simulink model "cmld_1m_vt"  (R2025b)
settings: Solver=ode23tb  StartTime=0.0  StopTime=12  MaxStep=5e-4  RelTol=1e-3
PreLoadFcn:
  | % --- generated CMLD self-contained defaults (cmld_params_for recipe, P=2405 MW baseline) ---
  | MotorA_Nom=[487413333.333333 11000 50]; MotorA_Stator=[0.02 0.072]; MotorA_Rotor=[0.05955 0.04937]; MotorA_Lm=1.728; MotorA_Mech=[0.1 0 2]; MotorA_Pmec=365560000; MotorA_Tm=0.786871368; MotorA_IC=[0.046858189966907 0 0 0 0 0 -120 120];
  | MotorB_Nom=[532306666.666667 11000 50]; MotorB_Stator=[0.03 0.114]; MotorB_Rotor=[0.0281 0.07959]; MotorB_Lm=1.686; MotorB_Mech=[0.5 0 2]; MotorB_Pmec=399230000; MotorB_Tm=0.7665097973; MotorB_IC=[0.0215389253032176 0 0 0 0 0 -120 120];
  | MotorC_Nom=[413660000 11000 50]; MotorC_Stator=[0.03 0.114]; MotorC_Rotor=[0.0281 0.07959]; MotorC_Lm=1.686; MotorC_Mech=[0.1 0 2]; MotorC_Pmec=310245000; MotorC_Tm=0.7665097973; MotorC_IC=[0.0215389253032176 0 0 0 0 0 -120 120];
  | CMLD_ElecP=810485000; P0=409480000; Q0=103896000; Pfrq=1.0;
  | CapC=0.037092; Fb_head=0.5;
undefined symbols (not defined in the file): dist_dP, dist_time, k_droop_f_g1, kt_hp, kt_lp, Lg_n1, M_g1, Motor_Tm, P_ref_g1, Rg_n1, Scc1, t_rh, theta_g0, Un1, Vpeak_g1, w_g1
libraries: spsControlledVoltageSourceLib x3, spsGroundLib x3, spsSeriesRLCBranchLib x3, spsThreePhaseParallelRLCBranchLib x2, spsThreePhaseParallelRLCLoadLib x1, spsThreePhaseSeriesRLCBranchLib x1, spsAsynchronousMachinepuUnitsLib x1, spsThreePhaseDynamicLoadLib x1, spsThreePhaseTransformerTwoWindingsLib x1, spsThreePhaseVIMeasurementLib x1, spspowerguiLib x1
settings Model: Creator=madeleineneaves  LastModifiedBy=madeleineneaves

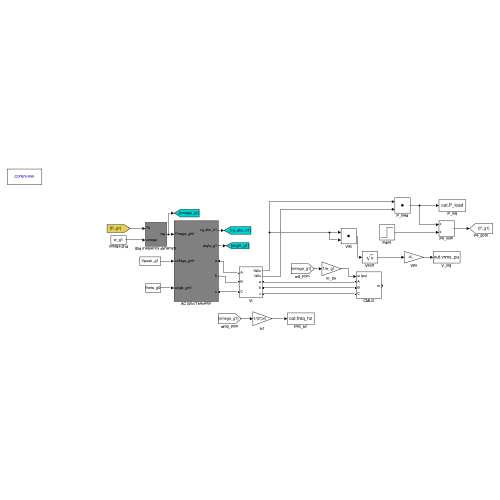
[thumbnail: Simulink's stored preview of the top-level diagram]
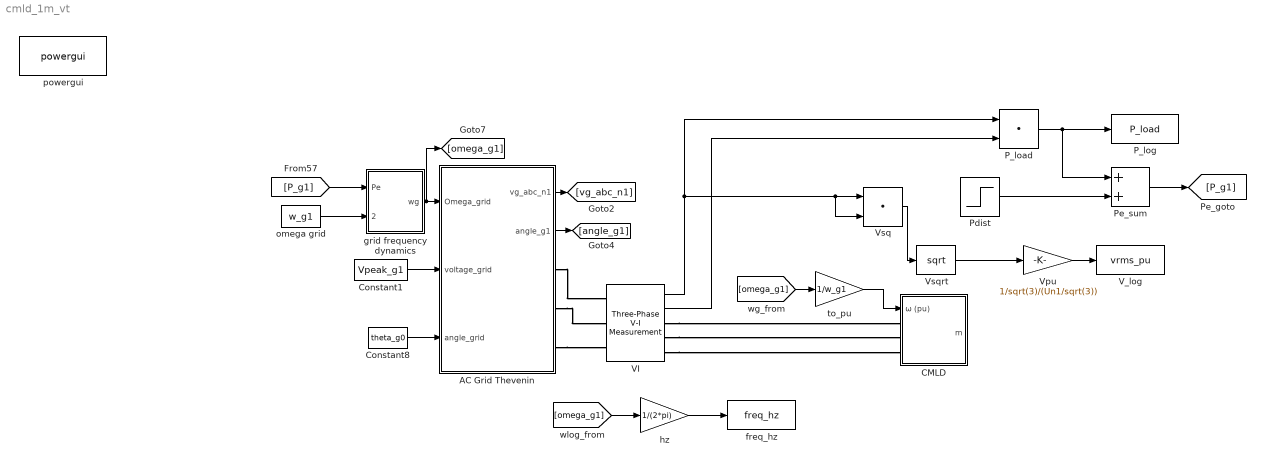
== system cmld_1m_vt ==
  AC Grid Thevenin : Subsystem
  CMLD : Subsystem
  Constant1 : Constant  Value=Vpeak_g1
  Constant8 : Constant  Value=theta_g0
  P_load : DotProduct  OutDataTypeStr=Inherit: Inherit via internal rule
  P_log : ToWorkspace  VariableName=P_load  SaveFormat=Timeseries  SampleTime=-1
  Pdist : Step  Time=dist_time  After=dist_dP  SampleTime=0
  Pe_sum : Sum
  VI : spsThreePhaseVIMeasurementLib/Three-Phase V-I Measurement  VoltageMeasurement=phase-to-ground  SetLabelV=off  LabelV=Vabc  Vpu=off  VpuLL=off  CurrentMeasurement=yes  SetLabelI=off  LabelI=Iabc  Ipu=off  Pbase=100e6  Vbase=500e3  OutputType=Complex  PhasorSimulation=off  PSBequivalent=0
  V_log : ToWorkspace  VariableName=vrms_pu  SaveFormat=Timeseries  SampleTime=-1
  Vpu : Gain  Gain=1/sqrt(3)/(Un1/sqrt(3))
  Vsq : DotProduct  OutDataTypeStr=Inherit: Inherit via internal rule
  Vsqrt : Sqrt
  freq_hz : ToWorkspace  VariableName=freq_hz  SaveFormat=Timeseries  SampleTime=-1
  grid frequency dynamics : Subsystem
  hz : Gain  Gain=1/(2*pi)
  omega grid : Constant  Value=w_g1
  powergui : spspowerguiLib/powergui  Priority=1  SimulationMode=Continuous  SampleTime=50e-6  frequency=60  Iterations=50  frequencyindice=60  Pbase=100e6  ErrMax=1e-4  UnitsV=kV  UnitsW=MW  buscounter=0  FunctionMessages=off  echomessages=off  EnableUseOfTLC=off  CurrentSourceSwitches=off  DisableSnubberDevices=off  DisableRonSwitches=off  DisableVfSwitches=off  DisplayEquations=off  AutomaticDiscreteSolvers=off  SolverType=Tustin/Backward Euler (TBE)  Interpol=off  ExternalGateDelay=off  methode=off  Ts=100  x0status=blocks  SPID=on  SwTol=0  HookPort=off  NonlinearTolerance=1e-4  nMaxIteration=100  ContinueOnMaxIteration=off  RestoreLinks=warning  ResistiveCurrentMeasurement=off  Frange=[0:2:500]  Ylog=off  Xlog=on  ShowGrid=off  save=off  variable=ZData  structure=0  ZoomFFT=off  StartTime=0.0  cycles=1  DisplayStyle=1  fundamental=60  FreqAxis=off  MaxFrequency=1000  frequencyindicesteady=1  RmsSteady=1  display=off
  to_pu : Gain  Gain=1/w_g1
  wires:
  AC Grid Thevenin/2(angle_g1) -> [angle_g1]
  Constant8/1 -> AC Grid Thevenin/3(angle_grid)
  Constant1/1 -> AC Grid Thevenin/2(voltage_grid)
  grid frequency dynamics/1(wg) -> [omega_g1], AC Grid Thevenin/1(Omega_grid)
  AC Grid Thevenin/1(vg_abc_n1) -> [vg_abc_n1]
  omega grid/1 -> grid frequency dynamics/2(omega)
  [P_g1] -> grid frequency dynamics/1(Pe)
  VI/1 -> Vsq/1, Vsq/2, P_load/1
  VI/2 -> P_load/2
  P_load/1 -> Pe_sum/1, P_log/1
  Pdist/1 -> Pe_sum/2
  Pe_sum/1 -> [P_g1]
  [omega_g1] -> to_pu/1
  to_pu/1 -> CMLD/1(ω (pu))
  [omega_g1] -> hz/1
  hz/1 -> freq_hz/1
  Vsq/1 -> Vsqrt/1
  Vsqrt/1 -> Vpu/1
  Vpu/1 -> V_log/1
  connections:
  AC Grid Thevenin/RConn1 -- VI/LConn1
  AC Grid Thevenin/RConn2 -- VI/LConn2
  AC Grid Thevenin/RConn3 -- VI/LConn3
  VI/RConn1 -- CMLD/LConn1
  VI/RConn2 -- CMLD/LConn2
  VI/RConn3 -- CMLD/LConn3

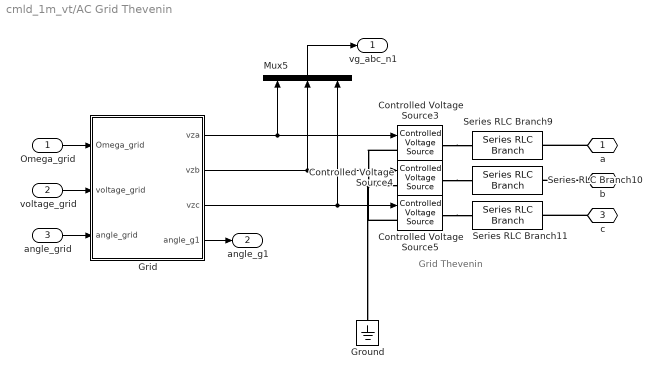
== system cmld_1m_vt/AC Grid Thevenin ==
  note: Grid Thevenin
  Omega_grid : Inport
  voltage_grid : Inport  Port=2
  angle_grid : Inport  Port=3
  Controlled Voltage Source3 : spsControlledVoltageSourceLib/Controlled Voltage Source  Initialize=on  Source_Type=AC  Amplitude=0  Phase=0  Frequency=0  Measurements=None
  Controlled Voltage Source4 : spsControlledVoltageSourceLib/Controlled Voltage Source  Initialize=on  Source_Type=AC  Amplitude=0  Phase=0  Frequency=0  Measurements=None
  Controlled Voltage Source5 : spsControlledVoltageSourceLib/Controlled Voltage Source  Initialize=on  Source_Type=AC  Amplitude=0  Phase=0  Frequency=0  Measurements=None
  Grid : Subsystem
  Ground : spsGroundLib/Ground  LConnTagsString=a
  Mux5 : Mux  Inputs=3
  Series RLC Branch10 : spsSeriesRLCBranchLib/Series RLC Branch  LConnTagsString=__new0  RConnTagsString=__new0  BranchType=RL  Resistance=Rg_n1  Inductance=Lg_n1  SetiL0=off  InitialCurrent=0  Capacitance=0  Setx0=off  InitialVoltage=0  Measurements=None
  Series RLC Branch11 : spsSeriesRLCBranchLib/Series RLC Branch  LConnTagsString=__new0  RConnTagsString=__new0  BranchType=RL  Resistance=Rg_n1  Inductance=Lg_n1  SetiL0=off  InitialCurrent=0  Capacitance=0  Setx0=off  InitialVoltage=0  Measurements=None
  Series RLC Branch9 : spsSeriesRLCBranchLib/Series RLC Branch  LConnTagsString=__new0  RConnTagsString=__new0  BranchType=RL  Resistance=Rg_n1  Inductance=Lg_n1  SetiL0=off  InitialCurrent=0  Capacitance=0  Setx0=off  InitialVoltage=0  Measurements=None
  a : PMIOPort  Side=Right
  b : PMIOPort  Port=2  Side=Right
  c : PMIOPort  Port=3  Side=Right
  vg_abc_n1 : Outport
  angle_g1 : Outport  Port=2
  wires:
  Mux5/1 -> vg_abc_n1/1
  Grid/1(vza) -> Mux5/1, Controlled Voltage Source3/1
  Grid/2(vzb) -> Controlled Voltage Source4/1, Mux5/2
  Grid/3(vzc) -> Mux5/3, Controlled Voltage Source5/1
  voltage_grid/1 -> Grid/2(voltage_grid)
  Omega_grid/1 -> Grid/1(Omega_grid)
  angle_grid/1 -> Grid/3(angle_grid)
  Grid/4(angle_g1) -> angle_g1/1
  connections:
  Controlled Voltage Source3/LConn1 -- Controlled Voltage Source4/LConn1 -- Ground/LConn1 -- Controlled Voltage Source5/LConn1
  Controlled Voltage Source3/RConn1 -- Series RLC Branch9/LConn1
  a/RConn1 -- Series RLC Branch9/RConn1
  Controlled Voltage Source4/RConn1 -- Series RLC Branch10/LConn1
  c/RConn1 -- Series RLC Branch11/RConn1
  Controlled Voltage Source5/RConn1 -- Series RLC Branch11/LConn1
  b/RConn1 -- Series RLC Branch10/RConn1

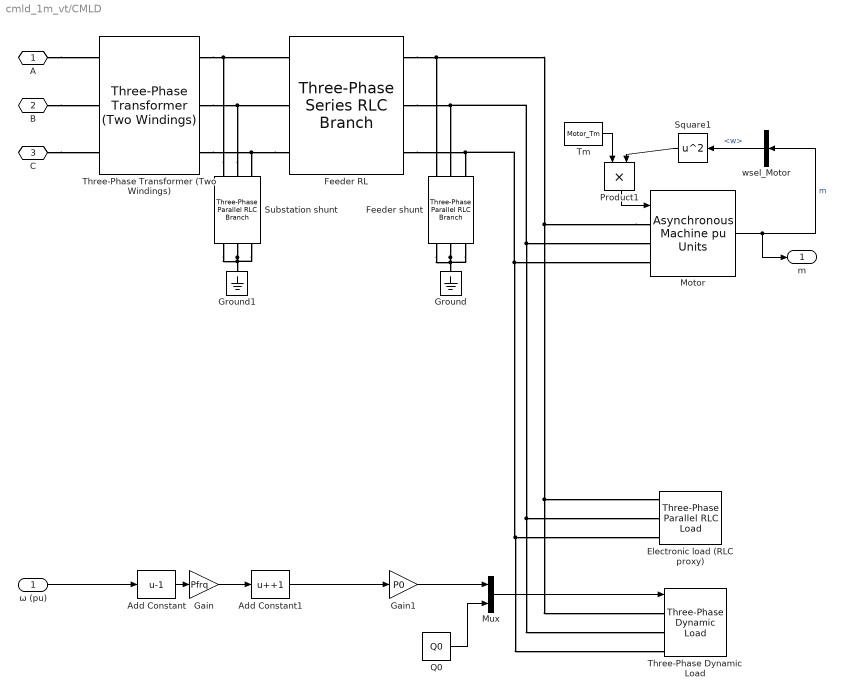
== system cmld_1m_vt/CMLD ==
  ω (pu) : Inport
  Add Constant : Bias  Bias=-1  SaturateOnIntegerOverflow=off
  Add Constant1 : Bias  Bias=+1  SaturateOnIntegerOverflow=off
  Electronic load (RLC proxy) : spsThreePhaseParallelRLCLoadLib/Three-Phase Parallel RLC Load  LConnTagsString=A|B|C  Configuration=Y (grounded)  NominalVoltage=11e3  Vabc=[1e3 1e3 1e3]  Vabcp=[1e3 1e3 1e3]  NominalFrequency=50  UnbalancedPower=off  ActivePower=CMLD_ElecP  InductivePower=0  CapacitivePower=0  Pabc=[10e3 9e3 11e3]  QLabc=[100 90 110]  QCabc=[100 90 110]  Pabcp=[10e3 9e3 11e3]  QLabcp=[100 90 110]  QCabcp=[100 90 110]  Measurements=None  LoadType=constant Z
  Feeder RL : spsThreePhaseSeriesRLCBranchLib/Three-Phase Series RLC Branch  LConnTagsString=A|B|C  RConnTagsString=A|B|C  BranchType=RL  Resistance=0.0002546  Inductance=1.8674e-05  Capacitance=1e-6  Measurements=None
  Feeder shunt : spsThreePhaseParallelRLCBranchLib/Three-Phase Parallel RLC Branch  LConnTagsString=A|B|C  RConnTagsString=A|B|C  BranchType=C  Resistance=1  Inductance=1e-3  Capacitance=CapC  Measurements=None
  Gain : Gain  Gain=Pfrq
  Gain1 : Gain  Gain=P0
  Ground : spsGroundLib/Ground  LConnTagsString=a
  Ground1 : spsGroundLib/Ground  LConnTagsString=a
  Motor : spsAsynchronousMachinepuUnitsLib/Asynchronous Machine pu Units  RotorType=Squirrel-cage  PresetModel=No  MechanicalLoad=Torque Tm  ShowDetailedParameters=on  ReferenceFrame=Rotor  Units=pu  MeasurementBus=on  NominalParameters=Motor_Nom  VoltageRatio=1  Stator=Motor_Stator  Rotor=Motor_Rotor  Cage1=[0.01909 0.0397]  Cage2=[0.01909 0.0397]  Lm=Motor_Lm  Mechanical=Motor_Mech  PolePairs=2  InitialConditions=Motor_IC  SimulateSaturation=off  Saturation="[0.212,0.4201,0.8125,1.0979,1.4799,2.2457,3.2586,4.5763,6.4763 ;   0.5,0.7,0.9,1,1.1,1.2 ,1.3,1.4,1.5]"  LoadFlowParameters=192400000  TsPowergui=0  TsBlock=-1  IterativeModel=Trapezoidal non iterative  IterativeDiscreteModel=Trapezoidal non iterative  Pmec=Motor_Pmec
      settings: LibrarySourceBlock=|
      | sps_lib/Electrical Machines/Asynchronous Machine
      | pu Units
  Mux : Mux  Inputs=2
  Product1 : Product
  Q0 : Constant  Value=Q0
  Square1 : Math  Operator=square
  Substation shunt : spsThreePhaseParallelRLCBranchLib/Three-Phase Parallel RLC Branch  LConnTagsString=A|B|C  RConnTagsString=A|B|C  BranchType=C  Resistance=1  Inductance=1e-3  Capacitance=CapC  Measurements=None
  Three-Phase Dynamic Load : spsThreePhaseDynamicLoadLib/Three-Phase Dynamic Load  NominalVoltage=[11e3 50]  ActiveReactivePowers=[50e6 25e6]  PositiveSequence=[0.994 -11.8]  ExternalControl=on  NpNq=[1.3 2]  TimeConstants="[0  0  0  0]"  MinimumVoltage=0.7  Tfilter=1e-4  LoadFlowParameters=[4,0,0,0,0]
      settings: LibrarySourceBlock=|
      | sps_lib/Passives/Three-Phase
      | Dynamic Load
  Three-Phase Transformer (Two Windings) : spsThreePhaseTransformerTwoWindingsLib/Three-Phase Transformer (Two Windings)  Winding1Connection=Yg  Winding2Connection=Yg  CoreType=Three single-phase transformers  SetSaturation=off  Hysteresis=off  DataFile='hysteresis'  SetInitialFlux=off  Measurements=None  UNITS=pu  NominalPower=[ 3000e6 , 50 ]  Winding1=[ 220e3 , 0.002 , 0.08 ]  Winding2=[ 11e3 , 0.002 , 0.08 ]  Rm=500  Lm=500  L0=0.5  Saturation=[ 0,0 ; 0.0024,1.2 ; 1.0,1.52 ]  InitialFluxes=[ 0.8 , -0.8 , 0.7 ]  BreakLoop=off  DiscreteSolver=Trapezoidal iterative  DataType=off  TransfoNumber=1
  Tm : Constant  Value=Motor_Tm
  wsel_Motor : BusSelector  OutputSignals=w
  A : PMIOPort  Side=Left
  B : PMIOPort  Port=2  Side=Left
  C : PMIOPort  Port=3  Side=Left
  m : Outport
  wires:
  Square1/1 -> Product1/2
  Tm/1 -> Product1/1
  Product1/1 -> Motor/1
  Motor/1 -> m/1, wsel_Motor/1  "m"
  Gain1/1 -> Mux/1
  Gain/1 -> Add Constant1/1
  ω (pu)/1 -> Add Constant/1
  Add Constant1/1 -> Gain1/1
  Mux/1 -> Three-Phase Dynamic Load/1
  Add Constant/1 -> Gain/1
  Q0/1 -> Mux/2
  wsel_Motor/1 -> Square1/1  "<w>"
  connections:
  Substation shunt/LConn2 -- Three-Phase Transformer (Two Windings)/RConn2 -- Feeder RL/LConn2
  Feeder shunt/RConn3 -- Feeder shunt/RConn2 -- Ground/LConn1 -- Feeder shunt/RConn1
  Substation shunt/LConn1 -- Three-Phase Transformer (Two Windings)/RConn1 -- Feeder RL/LConn1
  Feeder RL/LConn3 -- Three-Phase Transformer (Two Windings)/RConn3 -- Substation shunt/LConn3
  Substation shunt/RConn2 -- Substation shunt/RConn3 -- Substation shunt/RConn1 -- Ground1/LConn1
  Feeder RL/RConn2 -- Motor/LConn2 -- Electronic load (RLC proxy)/LConn2 -- Three-Phase Dynamic Load/LConn2 -- Feeder shunt/LConn2
  Motor/LConn1 -- Feeder shunt/LConn1 -- Feeder RL/RConn1 -- Electronic load (RLC proxy)/LConn1 -- Three-Phase Dynamic Load/LConn1
  Feeder RL/RConn3 -- Motor/LConn3 -- Three-Phase Dynamic Load/LConn3 -- Electronic load (RLC proxy)/LConn3 -- Feeder shunt/LConn3
  B/RConn1 -- Three-Phase Transformer (Two Windings)/LConn2
  A/RConn1 -- Three-Phase Transformer (Two Windings)/LConn1
  C/RConn1 -- Three-Phase Transformer (Two Windings)/LConn3

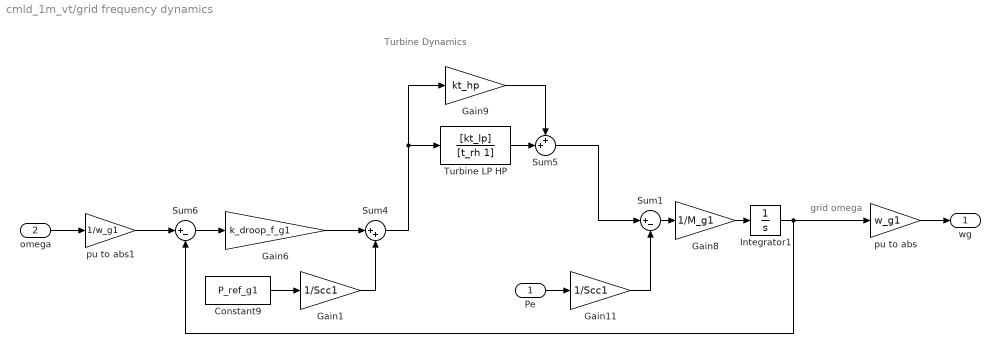
== system cmld_1m_vt/grid frequency dynamics ==
  note: Turbine Dynamics
  note: grid omega
  Pe : Inport
  omega : Inport  Port=2
  Constant9 : Constant  Value=P_ref_g1
  Gain1 : Gain  Gain=1/Scc1
  Gain11 : Gain  Gain=1/Scc1
  Gain6 : Gain  Gain=k_droop_f_g1
  Gain8 : Gain  Gain=1/M_g1
  Gain9 : Gain  Gain=kt_hp
  Integrator1 : Integrator  InitialCondition=1
  Sum1 : Sum  Inputs=|+-
  Sum4 : Sum  Inputs=|++
  Sum5 : Sum  Inputs=++|
  Sum6 : Sum  Inputs=|+-
  Turbine LP HP : TransferFcn  Numerator=[kt_lp]  Denominator=[t_rh 1]
  pu to abs : Gain  Gain=w_g1
  pu to abs1 : Gain  Gain=1/w_g1
  wg : Outport
  wires:
  pu to abs1/1 -> Sum6/1
  Gain9/1 -> Sum5/1
  Sum6/1 -> Gain6/1
  Sum1/1 -> Gain8/1
  Integrator1/1 -> pu to abs/1, Sum6/2
  Gain11/1 -> Sum1/2
  Turbine LP HP/1 -> Sum5/2
  Sum4/1 -> Gain9/1, Turbine LP HP/1
  Gain6/1 -> Sum4/1
  Gain8/1 -> Integrator1/1
  Pe/1 -> Gain11/1
  pu to abs/1 -> wg/1
  Sum5/1 -> Sum1/1
  Gain1/1 -> Sum4/2
  omega/1 -> pu to abs1/1
  Constant9/1 -> Gain1/1

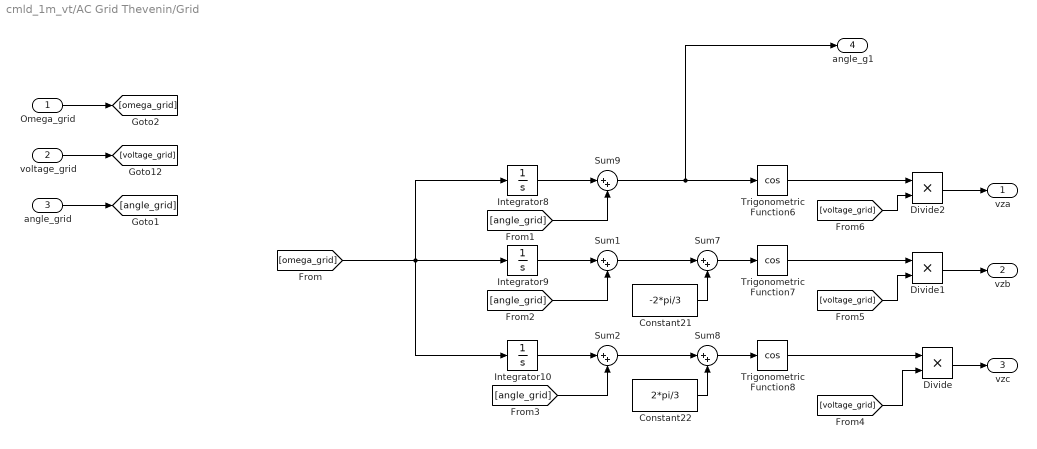
== system cmld_1m_vt/AC Grid Thevenin/Grid ==
  Omega_grid : Inport
  voltage_grid : Inport  Port=2
  angle_grid : Inport  Port=3
  Constant21 : Constant  Value=-2*pi/3
  Constant22 : Constant  Value=2*pi/3
  Divide : Product  Inputs=**
  Divide1 : Product  Inputs=**
  Divide2 : Product  Inputs=**
  Integrator10 : Integrator
  Integrator8 : Integrator
  Integrator9 : Integrator
  Sum{1..2,7..9} (5 alike) : Sum  Inputs=|++
  Trigonometric Function6 : Trigonometry  Operator=cos
  Trigonometric Function7 : Trigonometry  Operator=cos
  Trigonometric Function8 : Trigonometry  Operator=cos
  vza : Outport  VectorParamsAs1DForOutWhenUnconnected=off
  vzb : Outport  Port=2  VectorParamsAs1DForOutWhenUnconnected=off
  vzc : Outport  Port=3  VectorParamsAs1DForOutWhenUnconnected=off
  angle_g1 : Outport  Port=4  VectorParamsAs1DForOutWhenUnconnected=off
  wires:
  Trigonometric Function8/1 -> Divide/1
  Trigonometric Function7/1 -> Divide1/1
  Sum9/1 -> angle_g1/1, Trigonometric Function6/1
  Constant22/1 -> Sum8/2
  Sum2/1 -> Sum8/1
  Constant21/1 -> Sum7/2
  Integrator8/1 -> Sum9/1
  Sum7/1 -> Trigonometric Function7/1
  [angle_grid] -> Sum9/2
  Sum1/1 -> Sum7/1
  Sum8/1 -> Trigonometric Function8/1
  Trigonometric Function6/1 -> Divide2/1
  [voltage_grid] -> Divide/2
  Divide/1 -> vzc/1
  Divide1/1 -> vzb/1
  Divide2/1 -> vza/1
  Integrator9/1 -> Sum1/1
  angle_grid/1 -> [angle_grid]
  voltage_grid/1 -> [voltage_grid]
  Omega_grid/1 -> [omega_grid]
  [omega_grid] -> Integrator10/1, Integrator8/1, Integrator9/1
  [angle_grid] -> Sum1/2
  Integrator10/1 -> Sum2/1
  [angle_grid] -> Sum2/2
  [voltage_grid] -> Divide1/2
  [voltage_grid] -> Divide2/2
